simulink model "dead_beat_control"  (R2024b)
settings: Solver=ode1  StartTime=0.0  StopTime=2  FixedStep=1e-6  RelTol=1e-3
values from neighbouring files (symbols this model uses):
  V = VPH - mean(VPH)    [three_level_inverter.m]
libraries: eeGeneralControl x2, simulink x2, spsDCVoltageSourceLib x1, spsPermanentMagnetSynchronousMachineLib x1, spsThreePhaseVIMeasurementLib x1, spsUniversalBridgeLib x1, spsabctoAlphaBetaZeroLib x1, mcbcontrolslib x1, slpidlib x1, spsdq0toabcLib x1, spspowerguiLib x1
settings Model: SimulationMode=accelerator  Creator=killa  LastModifiedBy=killa
settings SolverCC: ZeroCrossAlgorithm=Adaptive
settings DebuggingCC: IgnoredZcDiagnostic=none

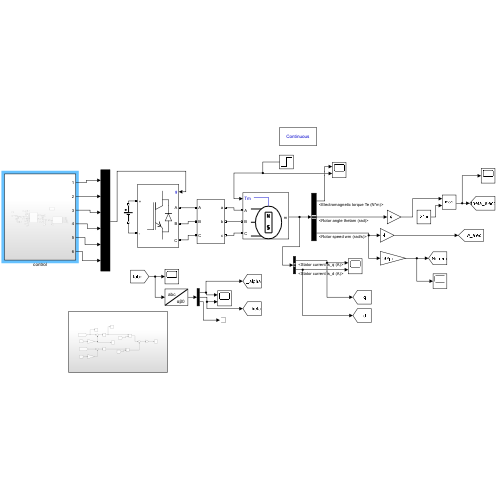
[thumbnail: Simulink's stored preview of the top-level diagram]
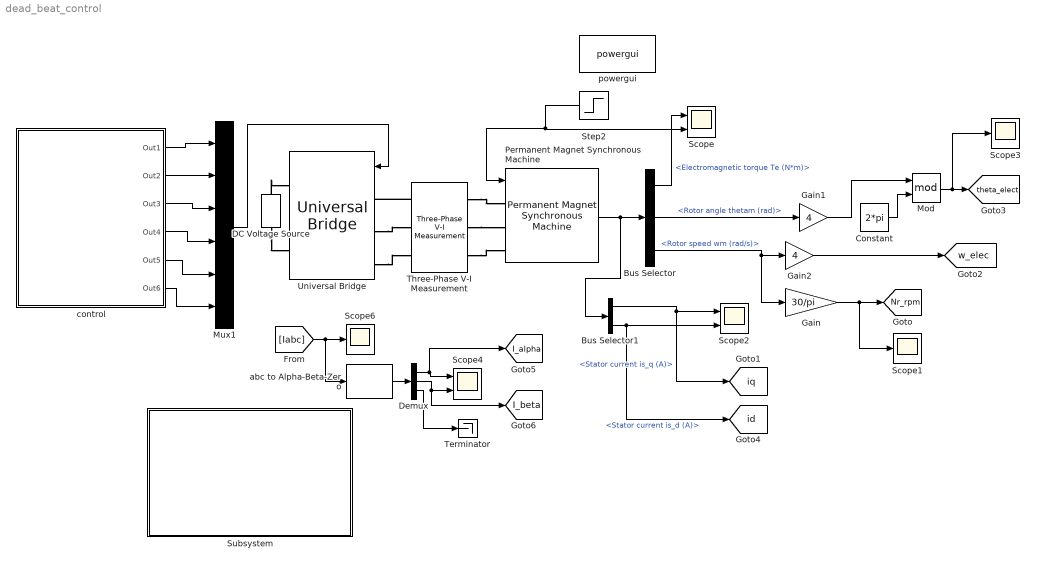
== system dead_beat_control ==
  Bus Selector : BusSelector  OutputSignals=Electromagnetic torque Te (N*m),Rotor angle thetam (rad),Rotor speed wm (rad/s)
  Bus Selector1 : BusSelector  OutputSignals=Stator current is_q (A),Stator current is_d (A)
  Constant : Constant  Value=2*pi
  DC Voltage Source : spsDCVoltageSourceLib/DC Voltage Source  Amplitude=300  Measurements=None
  Demux : Demux  Outputs=3
  Gain : Gain  Gain=30/pi
  Gain1 : Gain  Gain=4
  Gain2 : Gain  Gain=4
  Mod : Math  Operator=mod
  Mux1 : Mux  Inputs=6
  Permanent Magnet Synchronous Machine : spsPermanentMagnetSynchronousMachineLib/Permanent Magnet Synchronous Machine  NbPhases=3  FluxDistribution=Sinusoidal  RotorType=Round  MechanicalLoad=Torque Tm  PresetModel="05:  8 Nm 300 Vdc 2000 RPM - 10 Nm"  ShowDetailedParameters=on  MeasurementBus=off  Resistance=0.9585  Inductance=8.5e-3  dqInductances=[8.5e-3,8.5e-3]  La=0.00525  MachineConstant=Flux linkage established by magnets (V.s)  Flux=0.1827  VoltageCst=132.5525  TorqueCst=1.0962  Flat=120  Mechanical=[0.0006329 0.0003035 4 0]  PolePairs=4  InitialConditions=[0,0, 0,0]  InitialConditions5ph=[0 0 0 0 0 0]  RefAngle=Aligned with phase A axis (original Park)  IterativeDiscreteModel=Trapezoidal non iterative  TsBlock=-1  TsPowergui=0
  Scope : Scope  NumInputPorts=2
  Scope1 : Scope
  Scope2 : Scope  NumInputPorts=2
  Scope3 : Scope
  Scope4 : Scope  NumInputPorts=2
  Scope6 : Scope
  Step2 : Step  Before=2  After=7  SampleTime=0
  Subsystem : Subsystem
  Terminator : Terminator
  Three-Phase V-I Measurement : spsThreePhaseVIMeasurementLib/Three-Phase V-I Measurement  VoltageMeasurement=no  SetLabelV=on  LabelV=Vabc  Vpu=off  VpuLL=off  CurrentMeasurement=yes  SetLabelI=on  LabelI=Iabc  Ipu=off  Pbase=100e6  Vbase=500e3  OutputType=Complex  PhasorSimulation=off  PSBequivalent=0
  Universal Bridge : spsUniversalBridgeLib/Universal Bridge  Arms=3  SnubberResistance=1e5  SnubberCapacitance=inf  Device=IGBT / Diodes  Ron=1e-3  Lon=0  ForwardVoltages="[  0  0  ]"  ForwardVoltage=0  GTOparameters=[ 10e-6 , 20e-6 ]  IGBTparameters=[ 1e-6 , 2e-6 ]  Measurements=None  Measurements_2=None  converterType=Rectifier
  abc to Alpha-Beta-Zero : spsabctoAlphaBetaZeroLib/abc to Alpha-Beta-Zero
  control : Subsystem
  powergui : spspowerguiLib/powergui  Priority=1  SimulationMode=Continuous  SampleTime=50e-6  frequency=60  Iterations=50  frequencyindice=0  Pbase=100e6  ErrMax=1e-4  UnitsV=kV  UnitsW=MW  buscounter=0  FunctionMessages=off  echomessages=off  EnableUseOfTLC=off  CurrentSourceSwitches=off  DisableSnubberDevices=off  DisableRonSwitches=off  DisableVfSwitches=off  DisplayEquations=off  AutomaticDiscreteSolvers=off  SolverType=Tustin/Backward Euler (TBE)  Interpol=off  ExternalGateDelay=off  methode=off  Ts=100  x0status=blocks  SPID=on  SwTol=0  HookPort=off  NonlinearTolerance=1e-4  nMaxIteration=100  ContinueOnMaxIteration=off  RestoreLinks=warning  ResistiveCurrentMeasurement=off  Frange=[0:2:500]  Ylog=off  Xlog=on  ShowGrid=off  save=off  variable=ZData  structure=0  ZoomFFT=off  StartTime=0.0  cycles=1  DisplayStyle=1  fundamental=60  FreqAxis=off  MaxFrequency=1000  frequencyindicesteady=1  RmsSteady=1  display=off
  tag scope: I_alpha=global, I_beta=global, Nr_rpm=global, id=global, iq=global, theta_elect=global, w_elec=global
  wires:
  Bus Selector/1 -> Scope/1  "<Electromagnetic torque Te (N*m)>"
  Gain/1 -> Scope1/1, [Nr_rpm]
  Mux1/1 -> Universal Bridge/1
  Bus Selector/2 -> Gain1/1  "<Rotor angle thetam (rad)>"
  Bus Selector1/2 -> [id], Scope2/2  "<Stator current is_d (A)>"
  Bus Selector1/1 -> [iq], Scope2/1  "<Stator current is_q (A)>"
  Step2/1 -> Scope/2, Permanent Magnet Synchronous Machine/1
  Bus Selector/3 -> Gain/1, Gain2/1  "<Rotor speed wm (rad/s)>"
  Permanent Magnet Synchronous Machine/1 -> Bus Selector/1, Bus Selector1/1
  Gain2/1 -> [w_elec]
  control/1(Out1) -> Mux1/1
  control/2(Out2) -> Mux1/2
  control/3(Out3) -> Mux1/3
  control/4(Out4) -> Mux1/4
  control/5(Out5) -> Mux1/5
  control/6(Out6) -> Mux1/6
  Gain1/1 -> Mod/1
  Mod/1 -> Scope3/1, [theta_elect]
  Constant/1 -> Mod/2
  [Iabc] -> abc to Alpha-Beta-Zero/1, Scope6/1
  abc to Alpha-Beta-Zero/1 -> Demux/1
  Demux/1 -> [I_alpha], Scope4/1
  Demux/2 -> [I_beta], Scope4/2
  Demux/3 -> Terminator/1
  connections:
  Three-Phase V-I Measurement/RConn2 -- Permanent Magnet Synchronous Machine/LConn2
  Three-Phase V-I Measurement/RConn1 -- Permanent Magnet Synchronous Machine/LConn1
  DC Voltage Source/LConn1 -- Universal Bridge/RConn2
  Three-Phase V-I Measurement/RConn3 -- Permanent Magnet Synchronous Machine/LConn3
  DC Voltage Source/RConn1 -- Universal Bridge/RConn1
  Universal Bridge/LConn2 -- Three-Phase V-I Measurement/LConn2
  Three-Phase V-I Measurement/LConn1 -- Universal Bridge/LConn1
  Universal Bridge/LConn3 -- Three-Phase V-I Measurement/LConn3

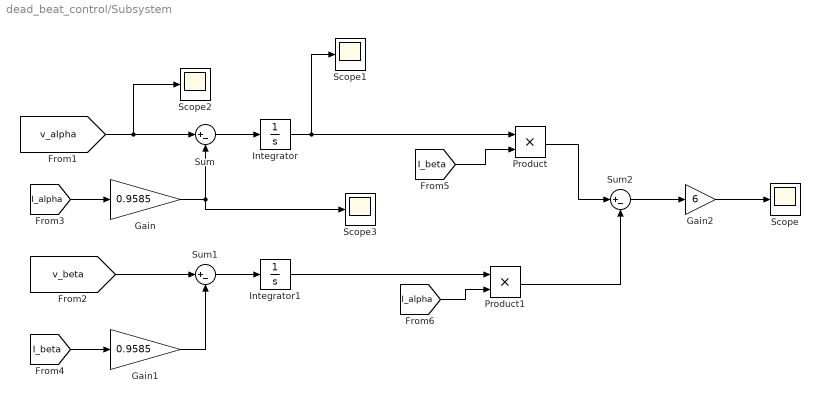
== system dead_beat_control/Subsystem ==
  Gain : Gain  Gain=0.9585
  Gain1 : Gain  Gain=0.9585
  Gain2 : Gain  Gain=6
  Integrator : Integrator
  Integrator1 : Integrator
  Product : Product
  Product1 : Product
  Scope{,1..3} (4 alike) : Scope
  Sum : Sum  Inputs=|+-
  Sum1 : Sum  Inputs=|+-
  Sum2 : Sum  Inputs=|+-
  wires:
  [v_alpha] -> Scope2/1, Sum/1
  [I_alpha] -> Gain/1
  Gain/1 -> Sum/2, Scope3/1
  Sum/1 -> Integrator/1
  [I_beta] -> Gain1/1
  [v_beta] -> Sum1/1
  Gain1/1 -> Sum1/2
  Sum1/1 -> Integrator1/1
  Integrator/1 -> Scope1/1, Product/1
  [I_beta] -> Product/2
  Integrator1/1 -> Product1/1
  [I_alpha] -> Product1/2
  Product/1 -> Sum2/1
  Product1/1 -> Sum2/2
  Sum2/1 -> Gain2/1
  Gain2/1 -> Scope/1

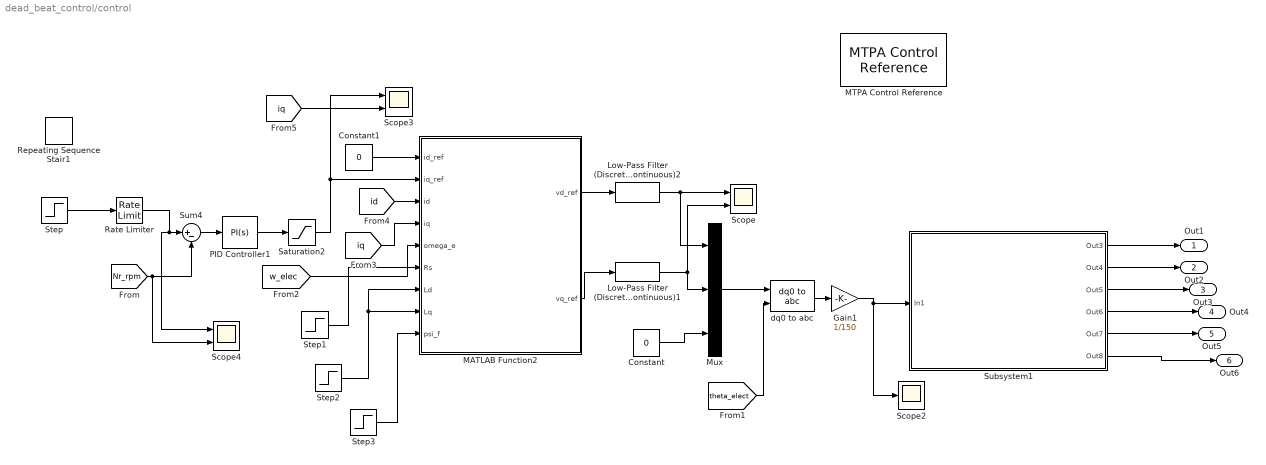
== system dead_beat_control/control ==
  Constant : Constant  Value=0
  Constant1 : Constant  Value=0
  Gain1 : Gain  Gain=1/150
  Low-Pass Filter (Discrete or Continuous)1 : eeGeneralControl/Low-Pass Filter (Discrete or Continuous)  K=1  T=318e-6  B=inf  A=-inf  init_option=Inherited from block input  x0=0  Ts=-1
  Low-Pass Filter (Discrete or Continuous)2 : eeGeneralControl/Low-Pass Filter (Discrete or Continuous)  K=1  T=318e-6  B=inf  A=-inf  init_option=Inherited from block input  x0=0  Ts=-1
  MATLAB Function2 : MATLAB Function  TreatAsAtomicUnit=on
  MTPA Control Reference : mcbcontrolslib/MTPA Control Reference  VariantSelect=Interior PMSM  polePairs=4  Rs=0.36  Ld=0.2e-3  Lq=0.4e-3  FluxPM=6.4e-3  ilimit=7.1  Vdc_input_select=Specify via dialog  V_dc=24  Units=Per-Unit (PU)  N_base=4107  I_base=19.3  T_base=0.74112  V_base=24/sqrt(3)  N_base_disp=3182  MTPAiterator=on  iterCount=10
      settings: LibrarySourceBlock=mcblib/Controls/Control Reference/MTPA Control Reference
  Mux : Mux  Inputs=3
  PID Controller1 : slpidlib/PID Controller  Controller=PI  Form=Parallel  TimeDomain=Continuous-time  UseExternalTs=off  SampleTime=-1  IntegratorMethod=Forward Euler  FilterMethod=Forward Euler  ControllerParametersSource=internal  P=0.1  I=1.5  UseKiTs=off  D=0  UseExternalDerivativeSource=off  N=100  UseFilter=on  TunerSelectOption=Transfer Function Based (PID Tuner App)  InitialConditionSource=internal  InitialConditionForIntegrator=0  InitialConditionForFilter=0  DifferentiatorICPrevScaledInput=0  ExternalReset=none  TrackingMode=off  Kt=1  LimitOutput=on  SatLimitsSource=internal  UpperSaturationLimit=inf  LowerSaturationLimit=-inf  LinearizeAsGain=on  AntiWindupMode=back-calculation  Kb=1.2/0.1  LimitIntegrator=off  UpperIntegratorSaturationLimit=inf  LowerIntegratorSaturationLimit=-inf  POutMin=[]  POutMax=[]  IOutMin=[]  IOutMax=[]  DOutMin=[]  DOutMax=[]  NOutMin=[]  NOutMax=[]  SumOutMin=[]  SumOutMax=[]  SaturationOutMin=[]  SaturationOutMax=[]  PParamMin=[]  PParamMax=[]  IParamMin=[]  IParamMax=[]  DParamMin=[]  DParamMax=[]  NParamMin=[]  NParamMax=[]  KbParamMin=[]  KbParamMax=[]  KtParamMin=[]  KtParamMax=[]  KbOutMin=[]  KbOutMax=[]  KtOutMin=[]  KtOutMax=[]  IntegratorOutMin=[]  IntegratorOutMax=[]  FilterOutMin=[]  FilterOutMax=[]  SumI1OutMin=[]  SumI1OutMax=[]  SumI2OutMin=[]  SumI2OutMax=[]  SumI3OutMin=[]  SumI3OutMax=[]  SumI4OutMin=[]  SumI4OutMax=[]  SumDOutMin=[]  SumDOutMax=[]  DifferentiatorOutMin=[]  DifferentiatorOutMax=[]  FilterDiffOutCoefMin=[]  FilterDiffOutCoefMax=[]  ReciprocalOutMin=[]  ReciprocalOutMax=[]  SumDenOutMin=[]  SumDenOutMax=[]  SumNumOutMin=[]  SumNumOutMax=[]  DivideOutMin=[]  DivideOutMax=[]  UdiffTsProdOutMin=[]  UdiffTsProdOutMax=[]  NTsProdOutMin=[]  NTsProdOutMax=[]  UintegralTsProdOutMin=[]  UintegralTsProdOutMax=[]  UngainTsProdOutMin=[]  UngainTsProdOutMax=[]  ClampingZeroOutDataTypeStr=Inherit: Inherit via back propagation  ClampingZeroOutMin=[]  ClampingZeroOutMax=[]  FilterDenConstantOutDataTypeStr=Inherit: Inherit via back propagation  FilterDenConstantOutMin=[]  FilterDenConstantOutMax=[]  PCopyOutDataTypeStr=Inherit: Inherit via back propagation  PCopyOutMin=[]  PCopyOutMax=[]  NCopyOutDataTypeStr=Inherit: Inherit via back propagation  NCopyOutMin=[]  NCopyOutMax=[]  IntegratorContinuousStateAttributes=''  IntegratorStateMustResolveToSignalObject=off  IntegratorRTWStateStorageClass=Auto  FilterContinuousStateAttributes=''  FilterStateMustResolveToSignalObject=off  FilterRTWStateStorageClass=Auto  ParallelPVariant=InternalParameters  IdealPVariant=Disabled  IVariant=InternalParameters  DVariant=Disabled  IntegratorVariant=Continuous  SatVariant=Enabled  AWVariant=BackCalculation  PCopyVariant=Disabled  TRVariant=Disabled  FdbkBlocksVariant=Forward  IdealPFdbkVariant=Disabled  SatFdbkVariant=Disabled  DerivativeFilterVariant=Disabled  NVariant=Disabled  NCopyVariant=Disabled_SignalSpec  FilterICVariant=Disabled  IntegratorICVariant=InternalICs  ExternalResetVariant=Disabled  TRSumVariant=Passthrough  SumFdbkVariant=Disabled  SumVariant=Sum_PI  TsampFilterVariant=InternalTs  TsampNgainVariant=Passthrough  TsampIntegralVariant=Disabled_SignalSpec  ExternalSaturationOutDataTypeStr=Inherit: Same as second input  DerivativeSourceVariant=Disabled  PreIntVariant=InternalPreInt
  Rate Limiter : RateLimiter  RisingSlewLimit=15000  FallingSlewLimit=-15000
  Repeating Sequence Stair1 : simulink/Sources/Repeating Sequence Stair  OutValues=[500 -1000 1500 2000 1500 1000 ].'  tsamp=1  OutMin=[]  OutMax=[]  OutDataTypeStr=double  OutputDataTypeScalingMode=double  OutDataType=fixdt(0,8)  ConRadixGroup=Best Precision: Vector-wise  OutScaling=2^-12
  Saturation2 : Saturate  UpperLimit=10  LowerLimit=-10
  Scope : Scope  NumInputPorts=2
  Scope2 : Scope
  Scope3 : Scope  NumInputPorts=2
  Scope4 : Scope  NumInputPorts=2
  Step : Step  Before=1000  After=2000  SampleTime=0
  Step1 : Step  Time=1.25  Before=0.9585  After=2*0.9585  SampleTime=0
  Step2 : Step  Time=1.4  Before=0.00525  After=2*0.00525  SampleTime=0
  Step3 : Step  Time=1.7  Before=0.1827  After=0.5*0.1827  SampleTime=0
  Subsystem1 : Subsystem
  Sum4 : Sum  Inputs=|+-
  dq0 to abc : spsdq0toabcLib/dq0 to abc  Alignment=Aligned with phase A axis
  Out1 : Outport
  Out2 : Outport  Port=2
  Out3 : Outport  Port=3
  Out4 : Outport  Port=4
  Out5 : Outport  Port=5
  Out6 : Outport  Port=6
  wires:
  [Nr_rpm] -> Sum4/2, Scope4/2
  Constant/1 -> Mux/3
  Mux/1 -> dq0 to abc/1
  [theta_elect] -> dq0 to abc/2
  Saturation2/1 -> Scope3/1, MATLAB Function2/2(iq_ref)
  Constant1/1 -> MATLAB Function2/1(id_ref)
  [iq] -> MATLAB Function2/4(iq)
  [id] -> MATLAB Function2/3(id)
  dq0 to abc/1 -> Gain1/1
  PID Controller1/1 -> Saturation2/1
  Sum4/1 -> PID Controller1/1
  [w_elec] -> MATLAB Function2/5(omega_e)
  Gain1/1 -> Scope2/1, Subsystem1/1(In1)
  Subsystem1/1(Out3) -> Out1/1
  Subsystem1/2(Out4) -> Out2/1
  Subsystem1/3(Out5) -> Out3/1
  Subsystem1/4(Out6) -> Out4/1
  Subsystem1/5(Out7) -> Out5/1
  Subsystem1/6(Out8) -> Out6/1
  Step/1 -> Rate Limiter/1
  Rate Limiter/1 -> Scope4/1, Sum4/1
  [iq] -> Scope3/2
  Step1/1 -> MATLAB Function2/6(Rs)
  MATLAB Function2/1(vd_ref) -> Low-Pass Filter (Discrete or Continuous)2/1
  MATLAB Function2/2(vq_ref) -> Low-Pass Filter (Discrete or Continuous)1/1
  Low-Pass Filter (Discrete or Continuous)2/1 -> Scope/1, Mux/1
  Low-Pass Filter (Discrete or Continuous)1/1 -> Mux/2, Scope/2
  Step2/1 -> MATLAB Function2/7(Ld), MATLAB Function2/8(Lq)
  Step3/1 -> MATLAB Function2/9(psi_f)

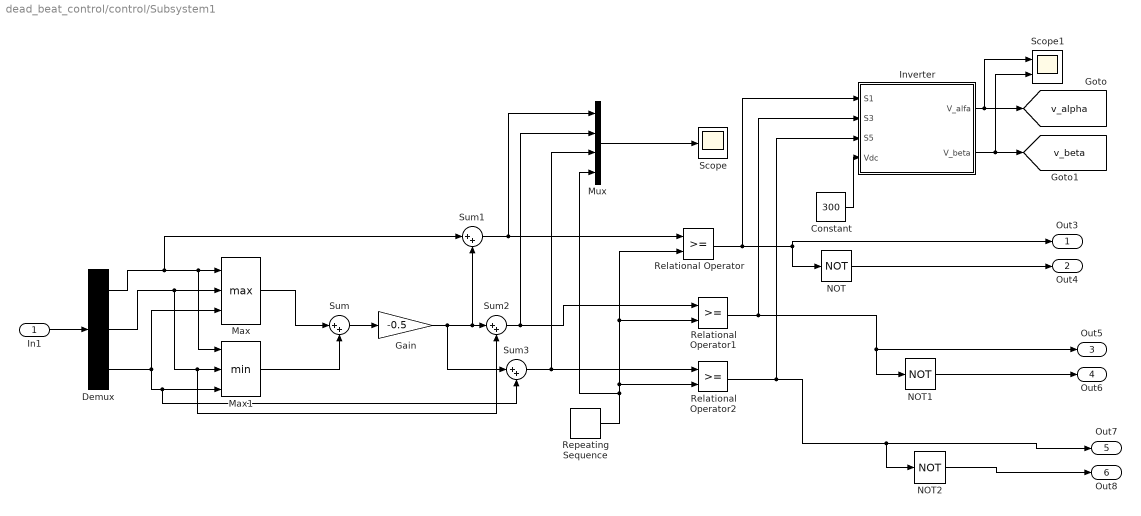
== system dead_beat_control/control/Subsystem1 ==
  In1 : Inport
  Constant : Constant  Value=300
  Demux : Demux  Outputs=3
  Gain : Gain  Gain=-0.5
  Inverter : Subsystem
  Max : MinMax  Function=max  Inputs=3
  Max1 : MinMax  Inputs=3
  Mux : Mux
  NOT : Logic  Operator=NOT  IconShape=distinctive  AllPortsSameDT=off  OutDataTypeStr=boolean
  NOT1 : Logic  Operator=NOT  IconShape=distinctive  AllPortsSameDT=off  OutDataTypeStr=boolean
  NOT2 : Logic  Operator=NOT  IconShape=distinctive  AllPortsSameDT=off  OutDataTypeStr=boolean
  Relational Operator : RelationalOperator  OutDataTypeStr=boolean  RndMeth=Simplest  InputSameDT=off
  Relational Operator1 : RelationalOperator  OutDataTypeStr=boolean  RndMeth=Simplest  InputSameDT=off
  Relational Operator2 : RelationalOperator  OutDataTypeStr=boolean  RndMeth=Simplest  InputSameDT=off
  Repeating Sequence : simulink/Sources/Repeating Sequence  rep_seq_t=[0 1 2]/20000  rep_seq_y=[-1 1 -1]
  Scope : Scope
  Scope1 : Scope  NumInputPorts=2
  Sum{,1..3} (4 alike) : Sum  Inputs=|++
  Out3 : Outport
  Out4 : Outport  Port=2
  Out5 : Outport  Port=3
  Out6 : Outport  Port=4
  Out7 : Outport  Port=5
  Out8 : Outport  Port=6
  tag scope: v_alpha=global, v_beta=global
  wires:
  Relational Operator2/1 -> Inverter/3(S5), Out7/1, NOT2/1
  NOT2/1 -> Out8/1
  NOT1/1 -> Out6/1
  Relational Operator1/1 -> Inverter/2(" S3 "), Out5/1, NOT1/1
  NOT/1 -> Out4/1
  Relational Operator/1 -> Inverter/1("S1 "), Out3/1, NOT/1
  In1/1 -> Demux/1
  Sum2/1 -> Mux/2, Relational Operator1/1
  Demux/1 -> Max/1, Max1/1, Sum1/1
  Demux/2 -> Max/2, Max1/2, Sum2/2
  Max1/1 -> Sum/2
  Sum3/1 -> Mux/3, Relational Operator2/1
  Max/1 -> Sum/1
  Sum/1 -> Gain/1
  Sum1/1 -> Mux/1, Relational Operator/1
  Gain/1 -> Sum3/1, Sum1/2, Sum2/1
  Demux/3 -> Max1/3, Sum3/2, Max/3
  Repeating Sequence/1 -> Mux/4, Relational Operator1/2, Relational Operator/2, Relational Operator2/2
  Mux/1 -> Scope/1
  Constant/1 -> Inverter/4(Vdc)
  Inverter/1(V_alfa) -> Scope1/1, [v_alpha]
  Inverter/2(V_beta) -> Scope1/2, [v_beta]

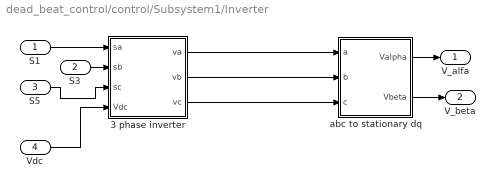
== system dead_beat_control/control/Subsystem1/Inverter ==
  "S1 " : Inport
  " S3 " : Inport  Port=2
  S5 : Inport  Port=3
  Vdc : Inport  Port=4
  3 phase inverter : Subsystem
  abc to stationary dq : Subsystem
  V_alfa : Outport
  V_beta : Outport  Port=2
  wires:
  abc to stationary dq/1(Valpha) -> V_alfa/1
  abc to stationary dq/2(Vbeta) -> V_beta/1
  "S1 "/1 -> 3 phase inverter/1(sa)
  " S3 "/1 -> 3 phase inverter/2(sb)
  S5/1 -> 3 phase inverter/3(sc)
  Vdc/1 -> 3 phase inverter/4(Vdc)
  3 phase inverter/1(va) -> abc to stationary dq/1(a)
  3 phase inverter/2(vb) -> abc to stationary dq/2(b)
  3 phase inverter/3(vc) -> abc to stationary dq/3(c)

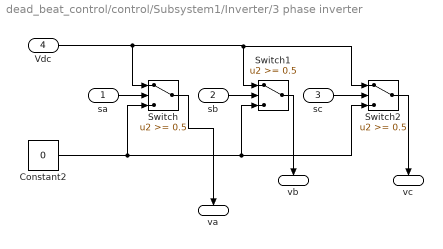
== system dead_beat_control/control/Subsystem1/Inverter/3 phase inverter ==
  sa : Inport
  sb : Inport  Port=2
  sc : Inport  Port=3
  Vdc : Inport  Port=4
  Constant2 : Constant  Value=0
  Switch : Switch  Threshold=0.5
  Switch1 : Switch  Threshold=0.5
  Switch2 : Switch  Threshold=0.5
  va : Outport  InitialOutput=0
  vb : Outport  Port=2  InitialOutput=0
  vc : Outport  Port=3  InitialOutput=0
  wires:
  Switch1/1 -> vb/1
  Switch2/1 -> vc/1
  sc/1 -> Switch2/2
  sb/1 -> Switch1/2
  sa/1 -> Switch/2
  Vdc/1 -> Switch2/1, Switch1/1, Switch/1
  Constant2/1 -> Switch/3, Switch1/3, Switch2/3
  Switch/1 -> va/1

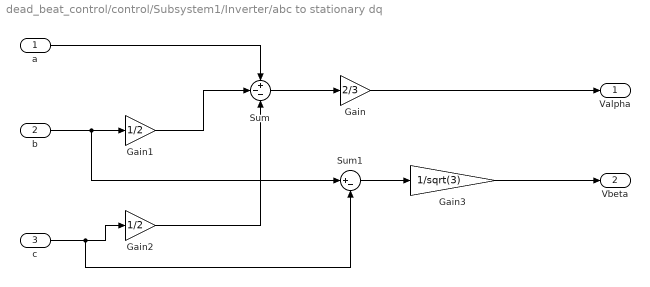
== system dead_beat_control/control/Subsystem1/Inverter/abc to stationary dq ==
  a : Inport
  b : Inport  Port=2
  c : Inport  Port=3
  Gain : Gain  Gain=2/3
  Gain1 : Gain  Gain=1/2
  Gain2 : Gain  Gain=1/2
  Gain3 : Gain  Gain=1/sqrt(3)
  Sum : Sum  Inputs=+--
  Sum1 : Sum  Inputs=|+-
  Valpha : Outport
  Vbeta : Outport  Port=2
  wires:
  a/1 -> Sum/1
  Sum/1 -> Gain/1
  c/1 -> Sum1/2, Gain2/1
  Sum1/1 -> Gain3/1
  Gain3/1 -> Vbeta/1
  Gain1/1 -> Sum/2
  b/1 -> Gain1/1, Sum1/1
  Gain2/1 -> Sum/3
  Gain/1 -> Valpha/1

== matlab function dead_beat_control/control/MATLAB Function2 ==
  settings: updateMethod=DISCRETE
  data: id_ref input; vd_ref output; iq_ref input; id input; iq input; omega_e input; vq_ref output; Rs input; Ld input; Lq input; psi_f input
function [vd_ref,vq_ref] = Deadbeat_Current_Controller(id_ref,iq_ref,id,iq,omega_e,Rs,Ld,Lq,psi_f)

% PMSM PARAMETERS
      % Ohm
      % Wb
Vdc   = 300;

% Sampling time
Ts = 1/20000;             % 100 us

%----------------------------------------------------------
% PERSISTENT STATE: voltage actually applied last sample
% (needed to compensate the 1-sample computation/PWM delay)
%----------------------------------------------------------
persistent vd_prev vq_prev
if isempty(vd_prev)
    vd_prev = 0;
    vq_prev = 0;
end

%----------------------------------------------------------
% ONE-STEP-AHEAD CURRENT PREDICTION
% Predict where id/iq will actually be when vd_prev/vq_prev
% (already in effect) finishes acting over this interval.
%----------------------------------------------------------
id_pred = id + (Ts/Ld)*(vd_prev - Rs*id + omega_e*Lq*iq);
iq_pred = iq + (Ts/Lq)*(vq_prev - Rs*iq - omega_e*(Ld*id + psi_f));

%----------------------------------------------------------
% CURRENT ERRORS (based on the PREDICTED state, not the
% raw measured one)
%----------------------------------------------------------
ed = id_ref - id_pred;
eq = iq_ref - iq_pred;

%----------------------------------------------------------
% DEADBEAT CURRENT CONTROL
%----------------------------------------------------------
vd_ref = Rs*id_pred + (Ld/Ts)*ed - omega_e*Lq*iq_pred;
vq_ref = Rs*iq_pred + (Lq/Ts)*eq + omega_e*(Ld*id_pred + psi_f);

%----------------------------------------------------------
% VOLTAGE LIMIT
%----------------------------------------------------------
Vmax = Vdc/sqrt(3);
Vmag = sqrt(vd_ref^2 + vq_ref^2);

if Vmag > Vmax
    vd_ref = vd_ref * Vmax/Vmag;
    vq_ref = vq_ref * Vmax/Vmag;
end
% Remember the voltage that will ACTUALLY be applied this
% sample (post-saturation!) so next call can predict correctly
vd_prev = vd_ref;
vq_prev = vq_ref;

end
